simulink model "BANSHEE"  (Simulink 8.7)
settings: Solver=ode1  StartTime=0.0  StopTime=inf  FixedStep=Ts  MaxStep=1e-3  RelTol=1e-3
PostLoadFcn:
  | BANSHEE_init;
InitFcn:
  | BANSHEE_init;
values from neighbouring files (symbols this model uses):
  Ts = 100E-6    (= 0.0001)    [BANSHEE_init.m]
undefined symbols (not defined in the file or in its folder): Acid, Banshee_HWCtrl_IOs, Banshee_SEL751_Woodward_lib, DMS_slave_lib, DMSCommands, F1, F2, F3, fdesignblkfcn, Feeder1_lib, Feeder2_lib, Feeder3_lib, gcbh, generic_ethernet_cb, Lead, Left, relay_housing_lib, SM_UtilityService, SS_F1_RELAY_HOUSING, SS_F2_RELAY_HOUSING, SS_F3_RELAY_HOUSING, SS_Feeder1, SS_Feeder2, SS_Feeder3, SUBSTATION, TestSeq_slave_lib, TestSequenceCommands, type, utility_service_lib, V
libraries: powerlib x108, cables_lib x61, breaker_lib x53, rtio_generic_modbus x50, relay_modbus_lib x45, rtio_opalrt_op5142ex1 x37, transformer_lib x29, rteventslib x28, Load_lib x25, simulink x24, rtlab x20, ssn_lib x19
(part 4 of 9)

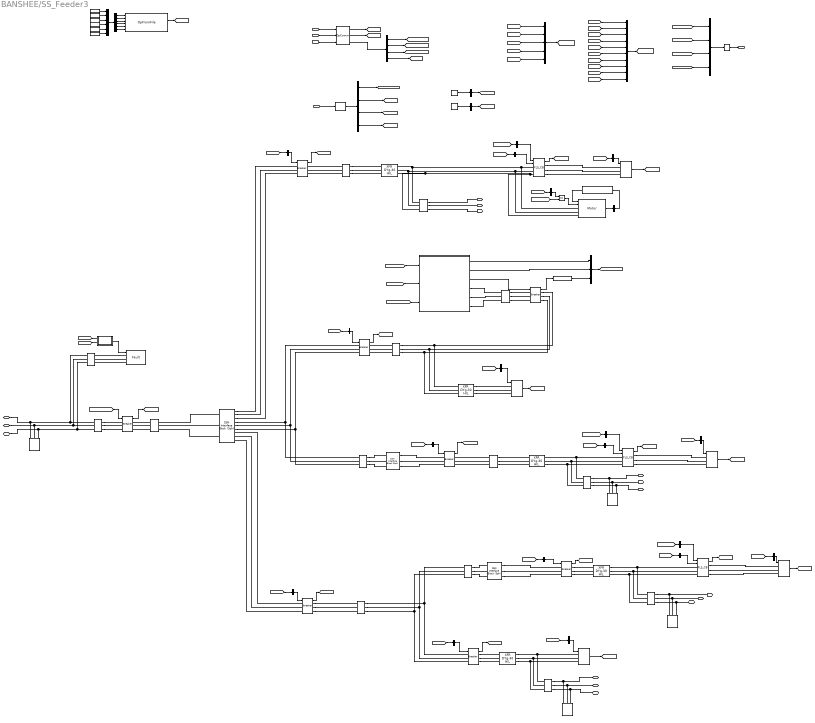
== system BANSHEE/SS_Feeder3 ==
  note: Signal for this Cb will come from a SEL relay
  note: connect to F2
  note: connect to F2
  note: connect to F2
  note: connect to F1
  note: % Copyright (c) 2016 Massachusetts Institute of Technology
      | % Permission is hereby granted, free of charge, to any person obtaining a copy of this
      | % software and associated documentation files (the "Software"), to deal in the Software
      | % without restriction, including without limitation the rights to use, copy, modify,
      | % merge, publish, distribute, sublicense, and/or sell copies of the Software, and to
      | % permit persons to whom the Software is furnished to do so, subject to the following
      | % conditions:
      | %
      | %
      | % The above copyright notice and this permission notice shall be included in
      | % all copies or substantial portions of the Software.
      | %
      | % THE SOFTWARE IS PROVIDED "AS IS", WITHOUT WARRANTY OF ANY KIND, EXPRESS OR IMPLIED,
      | % INCLUDING BUT NOT LIMITED TO THE WARRANTIES OF MERCHANTABILITY, FITNESS FOR A
      | % PARTICULAR PURPOSE AND NONINFRINGEMENT. IN NO EVENT SHALL THE AUTHORS OR COPYRIGHT
      | % HOLDERS BE LIABLE FOR ANY CLAIM, DAMAGES OR OTHER LIABILITY, WHETHER IN AN ACTION
      | % OF CONTRACT, TORT OR OTHERWISE, ARISING FROM, OUT OF OR IN CONNECTION WITH THE
      | % SOFTWARE OR THE USE OR OTHER DEALINGS IN THE SOFTWARE.
      | %
      | %
      | %%
  RELAY_IN : Inport
  LOAD_IN : Inport  Port=2
  SC_CMD : Inport  Port=3
  HWCtrl_CMD : Inport  Port=4
  1000 kVA : transformer_lib/XFR DYg-30 HIL  Rating=1000  Vp=13800  Vs=480  Z=5.75  XR=4.21
  1000 kVA1 : transformer_lib/XFR DYg-30 HIL  Rating=1000  Vp=13800  Vs=480  Z=5.75  XR=4.21
  200 HP chiller compressor : Load_lib/200 HP chiller compressor
  2000 kVA : transformer_lib/XFR DYg-30 HIL  Rating=2000  Vp=13800  Vs=480  Z=5.75  XR=4.7
  2000 kVA1 : transformer_lib/XFR DYg-30 HIL  Rating=2000  Vp=13800  Vs=480  Z=5.75  XR=4.7
  2500 kVA : transformer_lib/XFR DYg-30 HIL  Rating=2500  Vp=13800  Vs=480  Z=5.75  XR=6.6
  4/0AWG-Mutual : cables_lib/4//0AWG-Mutual  length=100  par_sets=1  ratio=3
  448 kvar inductor at 13.8kV  to cancel kvar produced by the stublines1 : powerlib/Elements/Three-Phase Parallel RLC Load  LConnTagsString=A|B|C  Configuration=Y (grounded)  NominalVoltage=13800  Vabc=[1e3 1e3 1e3]  Vabcp=[1e3 1e3 1e3]  NominalFrequency=60  UnbalancedPower=off  ActivePower=0  InductivePower=448e3  CapacitivePower=0  Pabc=[10e3 9e3 11e3]  QLabc=[100 90 110]  QCabc=[100 90 110]  Pabcp=[10e3 9e3 11e3]  QLabcp=[100 90 110]  QCabcp=[100 90 110]  Measurements=None  LoadType=constant Z
  500kcmil-Mutual{1..2,4,7} (4 alike) : cables_lib/500kcmil-Mutual  length=10  par_sets=1  ratio=3
  500kcmil-Mutual3 : cables_lib/500kcmil-Mutual  length=100  par_sets=1  ratio=3
  500kcmil-Mutual5 : cables_lib/500kcmil-Mutual  length=1000  par_sets=1  ratio=3
  500kcmil-Mutual9 : cables_lib/500kcmil-Mutual  length=1  par_sets=1  ratio=3
  6 kvar inductor at 480V  to cancel kvar produced by the stublines1 : powerlib/Elements/Three-Phase Parallel RLC Load  LConnTagsString=A|B|C  Configuration=Y (grounded)  NominalVoltage=480  Vabc=[1e3 1e3 1e3]  Vabcp=[1e3 1e3 1e3]  NominalFrequency=60  UnbalancedPower=off  ActivePower=0  InductivePower=6e3  CapacitivePower=0  Pabc=[10e3 9e3 11e3]  QLabc=[100 90 110]  QCabc=[100 90 110]  Pabcp=[10e3 9e3 11e3]  QLabcp=[100 90 110]  QCabcp=[100 90 110]  Measurements=None  LoadType=constant Z
  6 kvar inductor at 480V  to cancel kvar produced by the stublines2 : powerlib/Elements/Three-Phase Parallel RLC Load  LConnTagsString=A|B|C  Configuration=Y (grounded)  NominalVoltage=480  Vabc=[1e3 1e3 1e3]  Vabcp=[1e3 1e3 1e3]  NominalFrequency=60  UnbalancedPower=off  ActivePower=0  InductivePower=6e3  CapacitivePower=0  Pabc=[10e3 9e3 11e3]  QLabc=[100 90 110]  QCabc=[100 90 110]  Pabcp=[10e3 9e3 11e3]  QLabcp=[100 90 110]  QCabcp=[100 90 110]  Measurements=None  LoadType=constant Z
  6 kvar inductor at 480V  to cancel kvar produced by the stublines3 : powerlib/Elements/Three-Phase Parallel RLC Load  LConnTagsString=A|B|C  Configuration=Y (grounded)  NominalVoltage=480  Vabc=[1e3 1e3 1e3]  Vabcp=[1e3 1e3 1e3]  NominalFrequency=60  UnbalancedPower=off  ActivePower=0  InductivePower=6e3  CapacitivePower=0  Pabc=[10e3 9e3 11e3]  QLabc=[100 90 110]  QCabc=[100 90 110]  Pabcp=[10e3 9e3 11e3]  QLabcp=[100 90 110]  QCabcp=[100 90 110]  Measurements=None  LoadType=constant Z
  Bus Creator : BusCreator  Inputs=1
  Bus Creator1 : BusCreator  Inputs=1
  Bus Creator2 : BusCreator  Inputs=4
  Bus Creator3 : BusCreator  Inputs=5
  Bus Creator5 : BusCreator  Inputs=10
  Bus Creator6 : BusCreator  Inputs=3
  Bus Selector : BusSelector  OutputSignals=motor_2
  Bus Selector1 : BusSelector  OutputSignals=F3_CB_4
  Bus Selector10 : BusSelector  OutputSignals=F3_CB_5
  Bus Selector11 : BusSelector  OutputSignals=P6
  Bus Selector12 : BusSelector  OutputSignals=F3_CB_9
  Bus Selector13 : BusSelector  OutputSignals=F3_CB_3
  Bus Selector14 : BusSelector  OutputSignals=F3_CB_8
  Bus Selector15 : BusSelector  OutputSignals=IO ctrl.16 DOUT GR3.CHP_SIM_Cmds,motor_ONOFF.F3_motor_ONOFF,fault_cmd,GridStatusCtrl.Grid_F3.Logic_trip
  Bus Selector16 : BusSelector  OutputSignals=HWCtrl.NGCHP_Gen1,HWCtrl.SEL751_LogicTrip.F3.Logic_trip,HWCtrl.SEL2440_FLS,TestSeq
  Bus Selector17 : BusSelector  OutputSignals=RPM
  Bus Selector18 : BusSelector  OutputSignals=CB309
  Bus Selector19 : BusSelector  OutputSignals=CB307
  Bus Selector2 : BusSelector  OutputSignals=C6
  Bus Selector20 : BusSelector  OutputSignals=CB308
  Bus Selector3 : BusSelector  OutputSignals=P4
  Bus Selector4 : BusSelector  OutputSignals=I6
  Bus Selector5 : BusSelector  OutputSignals=C5
  Bus Selector6 : BusSelector  OutputSignals=F3_CB_2
  Bus Selector7 : BusSelector  OutputSignals=F3_CB_7
  Bus Selector8 : BusSelector  OutputSignals=F3_CB_6
  Bus Selector9 : BusSelector  OutputSignals=F3_CB_1
  C1 : cables_lib/500kcmil-Mutual  length=10  par_sets=1  ratio=3
  C2 : cables_lib/500kcmil-Mutual  length=10  par_sets=1  ratio=3
  C301 : cables_lib/500kcmil-Mutual  length=2500  par_sets=1  ratio=3
  C302 : cables_lib/4//0AWG-Mutual  length=2000  par_sets=1  ratio=3
  C303 : cables_lib/500kcmil-Mutual  length=2000  par_sets=1  ratio=3
  C304 : cables_lib/4//0AWG-Mutual  length=1500  par_sets=2  ratio=3
  CB closed : Constant
  CB open : Constant  Value=0
  Critical_5 : Load_lib/Dynamic_Load  V=480  kVA=1000  PF=0.9  Ts=Ts
  Critical_6 : Load_lib/Dynamic_Load  V=480  kVA=800  PF=0.9  Ts=Ts
  Demux2 : Demux  Outputs=6
  F3_CB_{1..6} (6 alike) : breaker_lib/Breaker  Ts=Ts  mech_delay=cb_mech_delay
  F3_CB_7 : breaker_lib/FLS_CB  Ts=Ts  mech_delay=cb_mech_delay
  F3_CB_8 : breaker_lib/FLS_CB  Ts=Ts  mech_delay=cb_mech_delay
  F3_CB_9 : breaker_lib/FLS_CB  Ts=Ts  mech_delay=cb_mech_delay
  F3_GCB : breaker_lib/Breaker  Ts=Ts  mech_delay=cb_mech_delay
  F3_PCC : breaker_lib/Breaker  Ts=Ts  mech_delay=cb_mech_delay
  Fault_4 : fault_lib/Fault  FaultResistance=0.1  GroundResistance=0.01  SnubberResistance=1E6
  HWController_3.5MVA_NGCHP : Subsystem  AncestorBlock=HWController_NGCHP_Genset_3p5MVA_lib/HWController_3.5MVA_NGCHP
  "Interpolation " : Constant
  Interruptible_6 : Load_lib/Dynamic_Load  V=480  kVA=600  PF=0.9  Ts=Ts
  Logical Operator : Logic  Operator=OR  AllPortsSameDT=off  OutDataTypeStr=boolean
  Memory : Memory
  Motor : Motor_InductionMachine_lib/Motor
  Mux : Mux  Inputs=6
  OpComm1 : rtlab/OpComm  nbport=3  groupe_acq=1  subsys_rate=0  st=0  Synchronization=on  Interpolation=on  Threshold=1.0  Missed_Data=off  Sim_Time=off  Samples=off  dynSigOut=off  from_console=0  warning_done=off  writeOpCommFile=off  Offset=off
  OpComm2 : rtlab/OpComm  nbport=1  groupe_acq=1  subsys_rate=0  st=0  Synchronization=on  Interpolation=on  Threshold=1.0  Missed_Data=off  Sim_Time=off  Samples=off  dynSigOut=off  from_console=1  warning_done=off  writeOpCommFile=off  Offset=off
  OpFromFile : rtlab/DataLogging/OpFromFile  filename_mode=Static (same filename all the time)  reload_mode=Next time model is paused (Real-Time)  init_file_id=0  filename=HeatLoad.mat  rtpath='./'  nrtpath='.\'  sample_time=Ts
  PQFV : PQFV_lib/PQFV  VRMSLL=13800  Ts=Ts
  Priority_4 : Load_lib/Dynamic_Load  V=480  kVA=600  PF=0.9  Ts=Ts
  Priority_6 : Load_lib/Dynamic_Load  V=480  kVA=1000  PF=0.9  Ts=Ts
  "Repetative " : Constant
  SSN Interface Block (3ph)1 : ssn_lib/SSN Interface Block (3ph)  nb_phase=3  nb_port=2  p1_type=V-type(Left)  p2_type=V-type (Right)  p3_type=V-type(Left)  p4_type=V-type(Left)  p5_type=V-type(Left)  p6_type=V-type(Left)  p7_type=V-type(Left)  p8_type=V-type(Left)  p9_type=V-type(Left)  p10_type=V-type(Left)  p11_type=V-type(Left)  p12_type=V-type(Left)  p13_type=V-type(Left)  p14_type=V-type(Left)  p15_type=V-type(Left)  p16_type=V-type(Left)  I_port_shunt_resistance=1e9
  SSN Interface Block (3ph)2 : ssn_lib/SSN Interface Block (3ph)  nb_phase=3  nb_port=2  p1_type=V-type(Left)  p2_type=V-type (Right)  p3_type=V-type(Left)  p4_type=V-type(Left)  p5_type=V-type(Left)  p6_type=V-type(Left)  p7_type=V-type(Left)  p8_type=V-type(Left)  p9_type=V-type(Left)  p10_type=V-type(Left)  p11_type=V-type(Left)  p12_type=V-type(Left)  p13_type=V-type(Left)  p14_type=V-type(Left)  p15_type=V-type(Left)  p16_type=V-type(Left)  I_port_shunt_resistance=1e9
  SSN Interface Block (3ph)5 : ssn_lib/SSN Interface Block (3ph)  nb_phase=3  nb_port=4  p1_type=V-type(Left)  p2_type=V-type (Right)  p3_type=V-type (Right)  p4_type=V-type (Right)  p5_type=V-type(Left)  p6_type=V-type(Left)  p7_type=V-type(Left)  p8_type=V-type(Left)  p9_type=V-type(Left)  p10_type=V-type(Left)  p11_type=V-type(Left)  p12_type=V-type(Left)  p13_type=V-type(Left)  p14_type=V-type(Left)  p15_type=V-type(Left)  p16_type=V-type(Left)  I_port_shunt_resistance=1e9
  "Start_Index " : Constant
  "State " : Constant
  "Stop_Index " : Constant  Value=1800-1
  "Time_Scale_Factor " : Constant
  fault_signal : Subsystem
  A_CB_4 : PMIOPort  Port=1  Side=Right
  B_CB_4 : PMIOPort  Port=2  Side=Right
  C_CB_4 : PMIOPort  Port=3  Side=Right
  A_CB_5 : PMIOPort  Port=4  Side=Right
  B_CB_5 : PMIOPort  Port=5  Side=Right
  C_CB_5 : PMIOPort  Port=6  Side=Right
  A_CB_6 : PMIOPort  Port=7  Side=Right
  B_CB_6 : PMIOPort  Port=8  Side=Right
  C_CB_6 : PMIOPort  Port=9  Side=Right
  A_CB_7 : PMIOPort  Port=10  Side=Right
  B_CB_7 : PMIOPort  Port=11  Side=Right
  C_CB_7 : PMIOPort  Port=12  Side=Right
  PCC_A : PMIOPort  Port=13  Side=Left
  PCC_B : PMIOPort  Port=14  Side=Left
  PCC_C : PMIOPort  Port=15  Side=Left
  DATA_OUT : Outport
  wires:
  CB closed/1 -> Bus Creator/1  "Logic_trip"
  Bus Creator/1 -> [cb_c]
  Bus Creator1/1 -> [cb_o]
  Bus Selector1/1 -> F3_CB_4/1  "<F3_CB_4>"
  CB open/1 -> Bus Creator1/1  "Logic_trip"
  LOAD_IN/1 -> OpComm1/1
  OpComm1/1 -> [LOAD_IN]
  [LOAD_IN] -> Bus Selector2/1
  [LOAD_IN] -> Bus Selector3/1
  [LOAD_IN] -> Bus Selector4/1
  [LOAD_IN] -> Bus Selector5/1
  Bus Selector2/1 -> Critical_6/1  "<C6>"
  Bus Selector3/1 -> Priority_4/1  "<P4>"
  Bus Selector4/1 -> Interruptible_6/1  "<I6>"
  Bus Selector5/1 -> Critical_5/1  "<C5>"
  Critical_6/1 -> [LOAD_C6]
  Priority_4/1 -> [LOAD_P4]
  Interruptible_6/1 -> [LOAD_I6]
  Critical_5/1 -> [LOAD_C5]
  [LOAD_C6] -> Bus Creator3/2  "F3_C6"
  [LOAD_C5] -> Bus Creator3/1  "F3_C5"
  [LOAD_I6] -> Bus Creator3/3  "F3_I6"
  [LOAD_P4] -> Bus Creator3/4  "F3_P4"
  Bus Creator3/1 -> [LOAD_DATA]  "LOAD"
  F3_CB_4/1 -> [F3_CB_4]
  F3_CB_3/1 -> [F3_CB_3]
  F3_CB_2/1 -> [F3_CB_2]
  F3_CB_6/1 -> [F3_CB_6]
  F3_CB_1/1 -> [F3_CB_1]
  F3_CB_5/1 -> [F3_CB_5]
  [F3_CB_1] -> Bus Creator5/1  "F3_CB_1"
  [F3_CB_5] -> Bus Creator5/5  "F3_CB_5"
  [F3_CB_7] -> Bus Creator5/7  "F3_CB_7"
  [F3_CB_6] -> Bus Creator5/6  "F3_CB_6"
  [F3_CB_3] -> Bus Creator5/3  "F3_CB_3"
  [F3_CB_2] -> Bus Creator5/2  "F3_CB_2"
  [F3_CB_4] -> Bus Creator5/4  "F3_CB_4"
  Bus Creator5/1 -> [CB_DATA]
  [RELAY_IN] -> Bus Selector1/1
  RELAY_IN/1 -> OpComm1/2
  OpComm1/2 -> [RELAY_IN]
  Bus Selector6/1 -> F3_CB_2/1  "<F3_CB_2>"
  [RELAY_IN] -> Bus Selector6/1
  Bus Selector7/1 -> F3_CB_7/2  "<F3_CB_7>"
  [RELAY_IN] -> Bus Selector7/1
  Bus Selector8/1 -> F3_CB_6/1  "<F3_CB_6>"
  [RELAY_IN] -> Bus Selector8/1
  Bus Selector9/1 -> F3_CB_1/1  "<F3_CB_1>"
  [RELAY_IN] -> Bus Selector9/1
  Bus Selector10/1 -> F3_CB_5/1  "<F3_CB_5>"
  [RELAY_IN] -> Bus Selector10/1
  Bus Selector13/1 -> F3_CB_3/1  "<F3_CB_3>"
  [RELAY_IN] -> Bus Selector13/1
  [SEL751_F3_LogicTrip] -> F3_PCC/1
  F3_CB_7/1 -> [F3_CB_7]
  F3_PCC/1 -> [F3_PCC]
  [F3_PCC] -> Bus Creator5/10  "F3_PCC"
  [LOAD_IN] -> Bus Selector11/1
  Bus Selector11/1 -> Priority_6/1  "<P6>"
  Priority_6/1 -> [LOAD_P6]
  [LOAD_P6] -> Bus Creator3/5  "F3_P6"
  F3_CB_9/1 -> [F3_CB_9]
  Bus Selector12/1 -> F3_CB_9/2  "<F3_CB_9>"
  [RELAY_IN] -> Bus Selector12/1
  F3_CB_8/1 -> [F3_CB_8]
  Bus Selector14/1 -> F3_CB_8/2  "<F3_CB_8>"
  [RELAY_IN] -> Bus Selector14/1
  [F3_CB_8] -> Bus Creator5/8  "F3_CB_8"
  [F3_CB_9] -> Bus Creator5/9  "F3_CB_9"
  SC_CMD/1 -> OpComm2/1
  Memory/1 -> DATA_OUT/1
  "Start_Index "/1 -> Mux/3
  "Time_Scale_Factor "/1 -> Mux/5
  "State "/1 -> Mux/1
  Demux2/1 -> OpFromFile/1
  Demux2/4 -> OpFromFile/4
  OpFromFile/2 -> [heat_load]  "Heat Load MBtu/hr"
  Demux2/5 -> OpFromFile/5
  "Repetative "/1 -> Mux/2
  Demux2/3 -> OpFromFile/3
  Demux2/6 -> OpFromFile/6
  Demux2/2 -> OpFromFile/2
  Mux/1 -> Demux2/1
  "Interpolation "/1 -> Mux/6
  "Stop_Index "/1 -> Mux/4
  Bus Selector15/2 -> [motor_cmd]  "<F3_motor_ONOFF>"
  OpComm2/1 -> Bus Selector15/1
  Bus Selector15/3 -> [fault_cmd]  "<fault_cmd>"
  F3_GCB/1 -> PQFV/1
  PQFV/1 -> Bus Creator6/3  "NG_CHP_GCB"
  HWController_3.5MVA_NGCHP/2(Generator Data) -> Bus Creator6/2  "Gen1_meas"
  HWController_3.5MVA_NGCHP/1(Out1) -> Bus Creator6/1  "CHPData"
  [CHP_SIM_cmds] -> HWController_3.5MVA_NGCHP/2(In2)
  Bus Creator6/1 -> [NG_CHP_DATA]
  [NGCHP_Gen1] -> HWController_3.5MVA_NGCHP/3(HWControllerBias)
  HWController_3.5MVA_NGCHP/3(GCB Control) -> F3_GCB/1
  [heat_load] -> HWController_3.5MVA_NGCHP/1(Heat Load MBtu/hrs)
  HWCtrl_CMD/1 -> OpComm1/3
  OpComm1/3 -> Bus Selector16/1
  Bus Selector16/1 -> [NGCHP_Gen1]  "<NGCHP_Gen1>"
  Bus Creator2/1 -> Memory/1
  [CB_DATA] -> Bus Creator2/1  "CB_DATA"
  [LOAD_DATA] -> Bus Creator2/2  "LOAD_DATA"
  [NG_CHP_DATA] -> Bus Creator2/3  "NG_CHP_DATA"
  Bus Selector15/1 -> [CHP_SIM_cmds]  "<CHP_SIM_Cmds>"
  Motor/1 -> Bus Selector17/1
  Bus Selector17/1 -> 200 HP chiller compressor/1  "<RPM>"
  200 HP chiller compressor/1 -> Motor/1
  [motor_cmd] -> Bus Creator2/4  "MOTOR_ONOFF"
  Bus Selector16/2 -> [SEL751_F3_LogicTrip]  "<Logic_trip>"
  Bus Selector16/3 -> [SEL_2440_FLS]  "<SEL2440_FLS>"
  [SEL_2440_FLS] -> Bus Selector18/1
  Bus Selector18/1 -> F3_CB_9/1  "<CB309>"
  [SEL_2440_FLS] -> Bus Selector19/1
  Bus Selector19/1 -> F3_CB_7/1  "<CB307>"
  [SEL_2440_FLS] -> Bus Selector20/1
  Bus Selector20/1 -> F3_CB_8/1  "<CB308>"
  Bus Selector15/4 -> [feeder_cb]  "<Logic_trip>"
  Bus Selector16/4 -> [TestSeq]  "<TestSeq>"
  [TestSeq] -> fault_signal/1(fault_ts)
  [fault_cmd] -> fault_signal/2(fault_sc)
  fault_signal/1(o) -> Fault_4/1
  [TestSeq] -> Bus Selector/1
  Logical Operator/1 -> Motor/2
  Bus Selector/1 -> Logical Operator/1  "<motor_2>"
  [motor_cmd] -> Logical Operator/2
  connections:
  C301/RConn1 -- C1/LConn1 -- F3_CB_5/LConn1
  F3_CB_6/RConn3 -- 2000 kVA1/LConn3
  C301/RConn3 -- C1/LConn3 -- F3_CB_5/LConn3
  C304/LConn1 -- F3_CB_2/RConn1
  F3_GCB/RConn3 -- C302/RConn3 -- 1000 kVA1/LConn3
  C302/LConn2 -- F3_CB_3/RConn2
  F3_GCB/RConn1 -- C302/RConn1 -- 1000 kVA1/LConn1
  F3_CB_6/RConn2 -- 2000 kVA1/LConn2
  F3_GCB/RConn2 -- C302/RConn2 -- 1000 kVA1/LConn2
  F3_CB_5/RConn2 -- 2000 kVA/LConn2
  C302/LConn3 -- F3_CB_3/RConn3
  C301/RConn2 -- C1/LConn2 -- F3_CB_5/LConn2
  C304/LConn2 -- F3_CB_2/RConn2
  F3_CB_6/RConn1 -- 2000 kVA1/LConn1
  C302/LConn1 -- F3_CB_3/RConn1
  F3_CB_5/RConn1 -- 2000 kVA/LConn1
  F3_CB_5/RConn3 -- 2000 kVA/LConn3
  C304/LConn3 -- F3_CB_2/RConn3
  F3_CB_7/RConn1 -- Priority_4/LConn1
  F3_CB_7/RConn3 -- Priority_4/LConn3
  F3_CB_7/RConn2 -- Priority_4/LConn2
  2000 kVA1/RConn1 -- 500kcmil-Mutual2/LConn1 -- F3_CB_8/LConn1
  500kcmil-Mutual2/LConn3 -- F3_CB_8/LConn3 -- 2000 kVA1/RConn3
  2000 kVA1/RConn2 -- 500kcmil-Mutual2/LConn2 -- F3_CB_8/LConn2
  2000 kVA/RConn1 -- 500kcmil-Mutual1/LConn1 -- Critical_5/LConn1
  2000 kVA/RConn3 -- 500kcmil-Mutual1/LConn3 -- Critical_5/LConn3
  2000 kVA/RConn2 -- 500kcmil-Mutual1/LConn2 -- Critical_5/LConn2
  Motor/LConn1 -- F3_CB_9/LConn1 -- 500kcmil-Mutual9/LConn1 -- 2500 kVA/RConn1
  F3_CB_9/LConn3 -- Motor/LConn3 -- 500kcmil-Mutual9/LConn3 -- 2500 kVA/RConn3
  Motor/LConn2 -- F3_CB_9/LConn2 -- 500kcmil-Mutual9/LConn2 -- 2500 kVA/RConn2
  C304/RConn2 -- 1000 kVA/LConn2
  C304/RConn3 -- 1000 kVA/LConn3
  C304/RConn1 -- 1000 kVA/LConn1
  F3_CB_7/LConn2 -- 500kcmil-Mutual4/LConn2 -- 1000 kVA/RConn2
  F3_CB_7/LConn1 -- 500kcmil-Mutual4/LConn1 -- 1000 kVA/RConn1
  F3_CB_9/RConn1 -- Priority_6/LConn1
  F3_CB_9/RConn2 -- Priority_6/LConn2
  F3_CB_9/RConn3 -- Priority_6/LConn3
  F3_CB_8/RConn1 -- Interruptible_6/LConn1
  F3_CB_8/RConn2 -- Interruptible_6/LConn2
  F3_CB_8/RConn3 -- Interruptible_6/LConn3
  SSN Interface Block (3ph)5/RConn1 -- F3_CB_4/LConn1
  SSN Interface Block (3ph)5/RConn3 -- F3_CB_4/LConn3
  SSN Interface Block (3ph)5/RConn2 -- F3_CB_4/LConn2
  SSN Interface Block (3ph)5/RConn4 -- F3_CB_3/LConn1 -- C2/LConn1
  SSN Interface Block (3ph)5/RConn6 -- F3_CB_3/LConn3 -- C2/LConn3
  SSN Interface Block (3ph)5/RConn5 -- C2/LConn2 -- F3_CB_3/LConn2
  C303/LConn1 -- F3_CB_4/RConn1
  C303/LConn2 -- F3_CB_4/RConn2
  C303/LConn3 -- F3_CB_4/RConn3
  C303/RConn2 -- 2500 kVA/LConn2
  C303/RConn3 -- 2500 kVA/LConn3
  C303/RConn1 -- 2500 kVA/LConn1
  Fault_4/LConn2 -- 500kcmil-Mutual7/RConn2
  Fault_4/LConn3 -- 500kcmil-Mutual7/RConn3
  Fault_4/LConn1 -- 500kcmil-Mutual7/RConn1
  4/0AWG-Mutual/RConn3 -- F3_GCB/LConn3
  4/0AWG-Mutual/RConn2 -- F3_GCB/LConn2
  4/0AWG-Mutual/RConn1 -- F3_GCB/LConn1
  HWController_3.5MVA_NGCHP/RConn2 -- 4/0AWG-Mutual/LConn2
  HWController_3.5MVA_NGCHP/RConn3 -- 4/0AWG-Mutual/LConn3
  HWController_3.5MVA_NGCHP/RConn1 -- 4/0AWG-Mutual/LConn1
  1000 kVA1/RConn1 -- Critical_6/LConn1
  1000 kVA1/RConn2 -- Critical_6/LConn2
  1000 kVA1/RConn3 -- Critical_6/LConn3
  500kcmil-Mutual1/RConn2 -- B_CB_5/RConn1 -- 6 kvar inductor at 480V  to cancel kvar produced by the stublines2/LConn2
  500kcmil-Mutual1/RConn1 -- 6 kvar inductor at 480V  to cancel kvar produced by the stublines2/LConn1 -- A_CB_5/RConn1
  500kcmil-Mutual1/RConn3 -- C_CB_5/RConn1 -- 6 kvar inductor at 480V  to cancel kvar produced by the stublines2/LConn3
  500kcmil-Mutual2/RConn2 -- 6 kvar inductor at 480V  to cancel kvar produced by the stublines1/LConn2 -- B_CB_6/RConn1
  500kcmil-Mutual2/RConn3 -- 6 kvar inductor at 480V  to cancel kvar produced by the stublines1/LConn3 -- C_CB_6/RConn1
  500kcmil-Mutual2/RConn1 -- 6 kvar inductor at 480V  to cancel kvar produced by the stublines1/LConn1 -- A_CB_6/RConn1
  500kcmil-Mutual4/RConn2 -- 6 kvar inductor at 480V  to cancel kvar produced by the stublines3/LConn2 -- B_CB_7/RConn1
  500kcmil-Mutual4/RConn3 -- 6 kvar inductor at 480V  to cancel kvar produced by the stublines3/LConn3 -- C_CB_7/RConn1
  500kcmil-Mutual4/RConn1 -- A_CB_7/RConn1 -- 6 kvar inductor at 480V  to cancel kvar produced by the stublines3/LConn1
  500kcmil-Mutual9/RConn1 -- A_CB_4/RConn1
  500kcmil-Mutual9/RConn3 -- C_CB_4/RConn1
  500kcmil-Mutual9/RConn2 -- B_CB_4/RConn1
  500kcmil-Mutual3/LConn3 -- F3_PCC/RConn3
  500kcmil-Mutual3/LConn1 -- F3_PCC/RConn1
  500kcmil-Mutual3/LConn2 -- F3_PCC/RConn2
  500kcmil-Mutual5/RConn1 -- F3_PCC/LConn1
  500kcmil-Mutual5/RConn2 -- F3_PCC/LConn2
  500kcmil-Mutual5/RConn3 -- F3_PCC/LConn3
  1000 kVA/RConn3 -- 500kcmil-Mutual4/LConn3 -- F3_CB_7/LConn3
  C1/RConn2 -- SSN Interface Block (3ph)1/LConn2
  C1/RConn3 -- SSN Interface Block (3ph)1/LConn3
  C1/RConn1 -- SSN Interface Block (3ph)1/LConn1
  SSN Interface Block (3ph)5/LConn1 -- 500kcmil-Mutual3/RConn1
  SSN Interface Block (3ph)5/LConn2 -- 500kcmil-Mutual3/RConn2
  SSN Interface Block (3ph)5/LConn3 -- 500kcmil-Mutual3/RConn3
  PCC_A/RConn1 -- 500kcmil-Mutual7/LConn1 -- 500kcmil-Mutual5/LConn1 -- 448 kvar inductor at 13.8kV  to cancel kvar produced by the stublines1/LConn1
  PCC_B/RConn1 -- 448 kvar inductor at 13.8kV  to cancel kvar produced by the stublines1/LConn2 -- 500kcmil-Mutual7/LConn2 -- 500kcmil-Mutual5/LConn2
  PCC_C/RConn1 -- 448 kvar inductor at 13.8kV  to cancel kvar produced by the stublines1/LConn3 -- 500kcmil-Mutual7/LConn3 -- 500kcmil-Mutual5/LConn3
  SSN Interface Block (3ph)2/RConn3 -- F3_CB_2/LConn3
  SSN Interface Block (3ph)2/RConn2 -- F3_CB_2/LConn2
  SSN Interface Block (3ph)2/RConn1 -- F3_CB_2/LConn1
  C2/RConn2 -- SSN Interface Block (3ph)2/LConn2
  C2/RConn1 -- SSN Interface Block (3ph)2/LConn1
  C2/RConn3 -- SSN Interface Block (3ph)2/LConn3
  F3_CB_1/LConn2 -- SSN Interface Block (3ph)5/RConn8
  F3_CB_1/LConn1 -- SSN Interface Block (3ph)5/RConn7
  F3_CB_1/LConn3 -- SSN Interface Block (3ph)5/RConn9
  SSN Interface Block (3ph)1/RConn1 -- F3_CB_6/LConn1
  SSN Interface Block (3ph)1/RConn2 -- F3_CB_6/LConn2
  SSN Interface Block (3ph)1/RConn3 -- F3_CB_6/LConn3
  F3_CB_1/RConn1 -- C301/LConn1
  F3_CB_1/RConn2 -- C301/LConn2
  F3_CB_1/RConn3 -- C301/LConn3

== system BANSHEE/SS_PV_BESS ==
  SC_CMD : Inport
  25% : Load_lib/Series_Constant_Load  v=480  kVA=1000  pf=0.9
  BESS : BESS_lib/BESS
  BESS Measurements : Subsystem
  Bus Creator6 : BusCreator  Inputs=2
  Bus Selector7 : BusSelector  OutputSignals=SWR_BESS,EPC_CTRL
  C1 : cables_lib/500kcmil-Mutual  length=10  par_sets=1  ratio=3
  C2 : cables_lib/500kcmil-Mutual  length=10  par_sets=1  ratio=3
  EPC : Subsystem
  Memory : Memory
  OpComm3 : rtlab/OpComm  nbport=1  groupe_acq=1  subsys_rate=0  st=0  Synchronization=on  Interpolation=on  Threshold=1.0  Missed_Data=off  Sim_Time=off  Samples=off  dynSigOut=off  from_console=1  warning_done=off  writeOpCommFile=off  Offset=off
  PV Measurements : Subsystem
  A_PV : PMIOPort  Port=1  Side=Right
  B_PV : PMIOPort  Port=2  Side=Right
  C_PV : PMIOPort  Port=3  Side=Right
  A_BESS : PMIOPort  Port=4  Side=Right
  B_BESS : PMIOPort  Port=5  Side=Right
  C_BESS : PMIOPort  Port=6  Side=Right
  BESS_PV : Outport
  wires:
  SC_CMD/1 -> OpComm3/1
  OpComm3/1 -> Bus Selector7/1
  Bus Selector7/1 -> [SWR_BESS]  "<SWR_BESS>"
  [SWR_BESS] -> BESS/1
  BESS/1 -> [BESS_MS]
  Memory/1 -> BESS_PV/1
  Bus Creator6/1 -> Memory/1
  [BESS_MS] -> Bus Creator6/1  "BESS"
  EPC/1(monitoring) -> [EPC_MS]
  [EPC_MS] -> Bus Creator6/2  "EPC"
  Bus Selector7/2 -> [EPC_CTRL]  "<EPC_CTRL>"
  [EPC_CTRL] -> EPC/1(FROM_SC)
  [EPC_MS] -> BESS Measurements/1(EPC_MS)
  [EPC_MS] -> PV Measurements/1(EPC_MS)
  connections:
  B_BESS/RConn1 -- C1/RConn2
  C_BESS/RConn1 -- C1/RConn3
  A_BESS/RConn1 -- C1/RConn1
  B_PV/RConn1 -- C2/RConn2
  C_PV/RConn1 -- C2/RConn3
  A_PV/RConn1 -- C2/RConn1
  EPC/LConn1 -- C1/LConn1
  EPC/LConn2 -- C1/LConn2
  EPC/LConn3 -- C1/LConn3
  EPC/LConn5 -- C2/LConn2
  EPC/LConn4 -- C2/LConn1
  EPC/LConn6 -- C2/LConn3
  25%/LConn2 -- BESS/RConn2
  25%/LConn3 -- BESS/RConn3
  25%/LConn1 -- BESS/RConn1

== system BANSHEE/SC_ctrl/EPC Inverter ==
  note: This corresponds to
      | the DIO Enable MCB
  note: Op_Mode:
      | 0 = Relay Functions
      | 1 = Close Breaker
      | 2 = Open Breaker
  16Din/16Dout GR3 : Subsystem
  16PWMIn/16PWMout GR3 : Subsystem
  16TSDIn/16 TSDOut GR3 : Subsystem
  Brk1 Grid : Constant  Value=2
  Brk10 Gen 1 Busbar : Constant
  Brk2 Load 1 : Constant  Value=0
  Brk3 Inv MX1 : Constant  Value=2
  Brk4 Gen 1 MCB : Constant  Value=2
  Brk5 Gen 2 LCB : Constant  Value=0
  Brk6 Gen 1 LCB : Constant  Value=0
  Brk7 Gen 2 GCB : Constant
  Brk8 Gen 1 GCB : Constant
  Brk9 Gen 2 Busbar : Constant
  Bus Creator1 : BusCreator  Inputs=3
  Bus Creator2 : BusCreator  Inputs=2
  Bus Creator3 : BusCreator  Inputs=14
  Wood MCB Enable : Constant  Value=0
  bias_ctrl : Constant
  control_mode : Constant
  gen_enable : Constant
  Out1 : Outport
  wires:
  Brk10 Gen 1 Busbar/1 -> Bus Creator3/10  "Gen1_Busbar"
  Brk9 Gen 2 Busbar/1 -> Bus Creator3/9  "Gen2_Busbar"
  Brk8 Gen 1 GCB/1 -> Bus Creator3/8  "Gen1_GCB"
  Brk7 Gen 2 GCB/1 -> Bus Creator3/7  "Gen2_GCB"
  Brk6 Gen 1 LCB/1 -> Bus Creator3/6  "Load 3"
  Brk5 Gen 2 LCB/1 -> Bus Creator3/5  "Load 2"
  Wood MCB Enable/1 -> Bus Creator3/14  "Wood_MCB_enable"
  Bus Creator2/1 -> Out1/1
  bias_ctrl/1 -> Bus Creator3/13  "Gen_bias_enable"
  gen_enable/1 -> Bus Creator3/12  "Gen2_enable"
  control_mode/1 -> Bus Creator3/11  "Wood_DIO"
  Brk4 Gen 1 MCB/1 -> Bus Creator3/4  "Gen1_MCB"
  Brk3 Inv MX1/1 -> Bus Creator3/3  "MX1"
  Brk2 Load 1/1 -> Bus Creator3/2  "Load 1"
  Brk1 Grid/1 -> Bus Creator3/1  "Grid"
  Bus Creator3/1 -> Bus Creator2/2  "test_controls"
  Bus Creator1/1 -> Bus Creator2/1  "DOUT GR3"
  16PWMIn/16PWMout GR3/1(To PWMOut) -> Bus Creator1/3  "16 PWMOUT GR3"
  16TSDIn/16 TSDOut GR3/1(TSDout) -> Bus Creator1/2  "16 TSDOUT GR3"
  16Din/16Dout GR3/1(Dout) -> Bus Creator1/1  "16 DOUT GR3"

== system BANSHEE/SC_ctrl/Inv_Battery ==
  note: Make this 1 to allow
      | the external signals.
  note: Remote Sense =>1
      | Use Remote Sense EPyQ
      | Sync or not => grid forming/grid following
  note: 0=> Local
      | 1=> Remote
  note: 0=> No Console
      | 1=> Console Ctrl
  note: 1 => Sig 1 is Bot then Sig 2 is Top
      | 0 => Sig 1 is Top then Sig 2 is Bot
  note: 0=> RTE
      | 1=> Simulink
  note: LSB
  note: MSB
  note: 1111: RTE TSD Signal Modulation External
      | 0111: RTE Signal Modulation Internal
      | X011: Sin Tri Modulatiion Internal
      | XX01: Digital Inputs
      | XXX0; Open Switches
  note: MCB
  note: GCB
  note: 1 => Closed
      | 0 => Open
  note: ~ 2.5 sec to get
      | to rated voltage
  note: RTE Internal
      | All 0 and one 1
  note: Internal = 0
      | External = 1
  Bus Creator : BusCreator  Inputs=8
  Bus Creator1 : BusCreator  Inputs=5
  Console : Constant  Value=0
  DC Contactor : Constant  Value=0
  Enable PWM{0..3} (4 alike) : Constant
  MX1 : Constant  Value=0
  MX2 : Constant  Value=0
  Precharge : Constant  Value=0
  Sense : Constant  Value=0
  Signal Mapping : Constant
  Simulink : Constant  Value=0
  S : Outport
  wires:
  Sense/1 -> Bus Creator/8  "LOCALvsREMOTE"
  Console/1 -> Bus Creator/7  "Console_Ctrl"
  Signal Mapping/1 -> Bus Creator1/5  "Ext_PWM_RTE_Signal"
  Simulink/1 -> Bus Creator/6  "RTEvsSPS"
  Enable PWM3/1 -> Bus Creator1/1
  Enable PWM2/1 -> Bus Creator1/2
  Enable PWM1/1 -> Bus Creator1/3
  Enable PWM0/1 -> Bus Creator1/4
  Bus Creator1/1 -> Bus Creator/1  "Enable PWM"
  MX2/1 -> Bus Creator/5  "MX2"
  MX1/1 -> Bus Creator/4  "MX1"
  DC Contactor/1 -> Bus Creator/3  "DC_Contactor"
  Precharge/1 -> Bus Creator/2  "Precharge"
  Bus Creator/1 -> S/1

== system BANSHEE/SC_ctrl/Inv_PV ==
  note: Make this 1 to allow
      | the external signals.
  note: Remote Sense =>1
      | Use Remote Sense EPyQ
      | Sync or not => grid forming/grid following
  note: 0=> Local
      | 1=> Remote
  note: 0=> No Console
      | 1=> Console Ctrl
  note: 1 => Sig 1 is Bot then Sig 2 is Top
      | 0 => Sig 1 is Top then Sig 2 is Bot
  note: 0=> RTE
      | 1=> Simulink
  note: LSB
  note: MSB
  note: 1111: RTE TSD Signal Modulation External
      | 0111: RTE Signal Modulation Internal
      | X011: Sin Tri Modulatiion Internal
      | XX01: Digital Inputs
      | XXX0; Open Switches
  note: MCB
  note: GCB
  note: 1 => Closed
      | 0 => Open
  note: ~ 2.5 sec to get
      | to rated voltage
  note: RTE Internal
      | All 0 and one 1
  note: Internal = 0
      | External = 1
  Bus Creator : BusCreator  Inputs=8
  Bus Creator1 : BusCreator  Inputs=5
  Console : Constant  Value=0
  DC Contactor : Constant  Value=0
  Enable PWM{0..3} (4 alike) : Constant
  MX1 : Constant  Value=0
  MX2 : Constant  Value=0
  Precharge : Constant  Value=0
  Sense : Constant  Value=0
  Signal Mapping : Constant
  Simulink : Constant  Value=0
  S : Outport
  wires:
  Sense/1 -> Bus Creator/8  "LOCALvsREMOTE"
  Console/1 -> Bus Creator/7  "Console_Ctrl"
  Signal Mapping/1 -> Bus Creator1/5  "Ext_PWM_RTE_Signal"
  Simulink/1 -> Bus Creator/6  "RTEvsSPS"
  Enable PWM3/1 -> Bus Creator1/1
  Enable PWM2/1 -> Bus Creator1/2
  Enable PWM1/1 -> Bus Creator1/3
  Enable PWM0/1 -> Bus Creator1/4
  Bus Creator1/1 -> Bus Creator/1  "Enable PWM"
  MX2/1 -> Bus Creator/5  "MX2"
  MX1/1 -> Bus Creator/4  "MX1"
  DC Contactor/1 -> Bus Creator/3  "DC_Contactor"
  Precharge/1 -> Bus Creator/2  "Precharge"
  Bus Creator/1 -> S/1

== system BANSHEE/SC_ctrl/Plots ==
  note: VRMSLL
      | Hz
      | kW
      | kVAR
  CMBNE_SGNLS : Inport
  Bus Selector1 : BusSelector  OutputSignals=F1_MS_IN.DIESEL_DATA.DIESEL_GCB.VRMSLL,F1_MS_IN.DIESEL_DATA.DIESEL_GCB.Freq,F1_MS_IN.DIESEL_DATA.DIESEL_GCB.kw,F1_MS_IN.DIESEL_DATA.DIESEL_GCB.kvar  OutputAsBus=on
  Bus Selector2 : BusSelector  OutputSignals=F3_MS_IN.NG_CHP_DATA.NG_CHP_GCB.VRMSLL,F3_MS_IN.NG_CHP_DATA.NG_CHP_GCB.Freq,F3_MS_IN.NG_CHP_DATA.NG_CHP_GCB.kw,F3_MS_IN.NG_CHP_DATA.NG_CHP_GCB.kvar  OutputAsBus=on
  Bus Selector3 : BusSelector  OutputSignals=PCC_DATA_OUT.F3_PCC.VRMSLL,PCC_DATA_OUT.F3_PCC.Freq,PCC_DATA_OUT.F3_PCC.kw,PCC_DATA_OUT.F3_PCC.kvar  OutputAsBus=on
  Bus Selector4 : BusSelector  OutputSignals=PCC_DATA_OUT.F2_PCC.VRMSLL,PCC_DATA_OUT.F2_PCC.Freq,PCC_DATA_OUT.F2_PCC.kw,PCC_DATA_OUT.F2_PCC.kvar  OutputAsBus=on
  Bus Selector5 : BusSelector  OutputSignals=PCC_DATA_OUT.F1_PCC.VRMSLL,PCC_DATA_OUT.F1_PCC.Freq,PCC_DATA_OUT.F1_PCC.kw,PCC_DATA_OUT.F1_PCC.kvar  OutputAsBus=on
  Bus Selector6 : BusSelector  OutputSignals=BESS_PV.EPC.PV.PV_MX1.VRMSLL,BESS_PV.EPC.PV.PV_MX1.Freq,BESS_PV.EPC.PV.PV_MX1.kw,BESS_PV.EPC.PV.PV_MX1.kvar  OutputAsBus=on
  Bus Selector7 : BusSelector  OutputSignals=BESS_PV.EPC.BESS.BESS_MX1.VRMSLL,BESS_PV.EPC.BESS.BESS_MX1.Freq,BESS_PV.EPC.BESS.BESS_MX1.kw,BESS_PV.EPC.BESS.BESS_MX1.kvar  OutputAsBus=on
  Bus Selector8 : BusSelector  OutputSignals=BESS_PV.EPC.BESS.BESS_MX1.cb_ms.Iabc,BESS_PV.EPC.BESS.BESS_MX1.cb_ms.Vabc_line,BESS_PV.EPC.PV.PV_MX1.cb_ms.Iabc,BESS_PV.EPC.PV.PV_MX1.cb_ms.Vabc_line
  Bus Selector9 : BusSelector  OutputSignals=SUBS_RELAY_OUT.SUBSTATION_CB_F1.m.status,SUBS_RELAY_OUT.SUBSTATION_CB_F2.m.status,SUBS_RELAY_OUT.SUBSTATION_CB_F3.m.status,SUBS_RELAY_OUT.SUBSTATION_CB_F1.Logic_trip,SUBS_RELAY_OUT.SUBSTATION_CB_F2.Logic_trip,SUBS_RELAY_OUT.SUBSTATION_CB_F3.Logic_trip  OutputAsBus=on
  CHP : Display
  Diesel : Display
  EPC_BESS : Display
  EPC_PV : Display
  F1 : Display
  F2 : Display
  F3 : Display
  SUBSTATION : Display
  Scope : Scope  NumInputPorts=4
  wires:
  Bus Selector5/1 -> F1/1
  Bus Selector4/1 -> F2/1
  Bus Selector3/1 -> F3/1
  Bus Selector1/1 -> Diesel/1
  Bus Selector2/1 -> CHP/1
  CMBNE_SGNLS/1 -> [CMBNE_SGNLS]
  [CMBNE_SGNLS] -> Bus Selector5/1
  [CMBNE_SGNLS] -> Bus Selector4/1
  [CMBNE_SGNLS] -> Bus Selector3/1
  [CMBNE_SGNLS] -> Bus Selector2/1
  [CMBNE_SGNLS] -> Bus Selector1/1
  [CMBNE_SGNLS] -> Bus Selector8/1, Bus Selector6/1
  Bus Selector6/1 -> EPC_PV/1
  [CMBNE_SGNLS] -> Bus Selector7/1
  Bus Selector7/1 -> EPC_BESS/1
  Bus Selector8/1 -> Scope/1  "<Iabc>"
  Bus Selector8/4 -> Scope/4  "<Vabc_line>"
  Bus Selector8/2 -> Scope/2  "<Vabc_line>"
  Bus Selector8/3 -> Scope/3  "<Iabc>"
  Bus Selector9/1 -> SUBSTATION/1
  [CMBNE_SGNLS] -> Bus Selector9/1

== system BANSHEE/SC_ctrl/TestSeq ==
  TestData : Inport
  Bus Selector : BusSelector  OutputSignals=TestSeq.TimeStamp,TestSeq.fault_location_1,TestSeq.fault_location_2,TestSeq.fault_location_3,TestSeq.fault_location_4,TestSeq.fault_location_5,TestSeq.Cut_Grid_Power,TestSeq.Irradiance,TestSeq.motor_1,TestSeq.motor_2,TestSeq.Test3
  Display : Display
  Scope : Scope  NumInputPorts=10
  wires:
  TestData/1 -> Bus Selector/1
  Bus Selector/1 -> Display/1  "<TimeStamp>"
  Bus Selector/6 -> Scope/5  "<fault_location_5>"
  Bus Selector/5 -> Scope/4  "<fault_location_4>"
  Bus Selector/10 -> Scope/9  "<motor_2>"
  Bus Selector/2 -> Scope/1  "<fault_location_1>"
  Bus Selector/3 -> Scope/2  "<fault_location_2>"
  Bus Selector/8 -> Scope/7  "<Irradiance>"
  Bus Selector/9 -> Scope/8  "<motor_1>"
  Bus Selector/4 -> Scope/3  "<fault_location_3>"
  Bus Selector/7 -> Scope/6  "<Cut_Grid_Power>"
  Bus Selector/11 -> Scope/10  "<Test3>"

== system BANSHEE/SC_ctrl/Woodward ==
  16Din/16Dout GR3 : Subsystem
  Bus Creator2 : BusCreator  Inputs=1
  IOctrl : Outport
  wires:
  16Din/16Dout GR3/1(Dout) -> Bus Creator2/1  "16 DOUT GR3"
  Bus Creator2/1 -> IOctrl/1  "IO ctrl"

== system BANSHEE/SM_UtilityService/Banshee_HWCtrl_IOs ==
  note: When the system uses the simulated
      | Secondary Controller the digital I/O
      | should be disabled.
  note: Copyright (c) 2016 Massachusetts Institute of Technology
      | Permission is hereby granted, free of charge, to any person obtaining a copy of this software and associated documentation files (the "Software"), to deal
      | in the Software without restriction, including without limitation the rights to use, copy, modify, merge, publish, distribute, sublicense, and/or sell copies of the
      | Software, and to permit persons to whom the Software is furnished to do so, subject to the following conditions:
      |
      | THE SOFTWARE IS PROVIDED "AS IS", WITHOUT WARRANTY OF ANY KIND, EXPRESS OR IMPLIED, INCLUDING BUT NOT LIMITED TO THE
      | WARRANTIES OF MERCHANTABILITY, FITNESS FOR A PARTICULAR PURPOSE AND NONINFRINGEMENT. IN NO EVENT SHALL THE AUTHORS
      | OR COPYRIGHT HOLDERS BE LIABLE FOR ANY CLAIM, DAMAGES OR OTHER LIABILITY, WHETHER IN AN ACTION OF CONTRACT, TORT OR
      | OTHERWISE, ARISING FROM, OUT OF OR IN CONNECTION WITH THE SOFTWARE OR THE USE OR OTHER DEALINGS IN THE SOFTWARE
  note: USE NEW  BITSTREAM
      | To use old bitstream, change Digital Output Channel from 13 to 9 inside
      | "SEL751_01_DigitalAnalog_IO_OpBlocks" block
  ScaledSignals : Inport
  CMBNE_SGNLS : Inport  Port=2
  DTT_like_Signal : Inport  Port=3
  Bus Creator : BusCreator  Inputs=4
  Bus Creator1 : BusCreator  Inputs=5
  Bus Creator2 : BusCreator  Inputs=5
  Bus Creator3 : BusCreator  Inputs=4
  Bus Selector1 : BusSelector  OutputSignals=MCB_CB_Status
  Bus Selector2 : BusSelector  OutputSignals=scaled_gcb_voltage,scaled_gcb_current,scaled_mcb_voltage,scaled_mcb_current,scaled_speed
  Bus Selector3 : BusSelector  OutputSignals=NGCHP_ScaledSignals,Diesel_ScaledSignals,SEL751_ScaledSignals
  Bus Selector4 : BusSelector  OutputSignals=scaled_gcb_voltage,scaled_gcb_current,scaled_mcb_voltage,scaled_mcb_current,scaled_speed
  Bus Selector5 : BusSelector  OutputSignals=MCB_CB_Status
  Demux1 : Demux  Outputs=16
  GR1 B AIN (CH00-15) : Subsystem
  Memory1 : Memory
  OP5142EX1 Ctrl : rtio_opalrt_op5142ex1/OpCtrl OP5142EX1  CtrlName='OP5142EX1 Ctrl'  boardid=1  BitstreamFilename=OP5142_1-EX-0000-2_3_5_87-16AI_48AO_32DIO_16DO_16selDO_CD-FF-01.bin  numconfig=-1  mode=Slave  externalClock=off  decimRtsi=0  calibIO=off  SampleTime=0  loadinport=-1
  OpCtrl : rtio_opalrt_common/OpCtrl  CtrlName='OpCtrl'  boardid=0  BitstreamFilename=VC707_2-EX-0001-2_3_2_20-48AIO16DIO16DIOSel-02-01.bin  numconfig=-1  mode=Master  externalClock=off  decimRtsi=0  calibIO=off  SampleTime=0  loadinport=-1  BoardType=VC707  SecondaryPresent=off  sync_type=Audio
  SEL-2440 FAST-LOAD-SHEDDING AND CB STATUS : Subsystem
  SEL751_DigitalAnalog_IO_OpBlocks : Subsystem
  Woodward Inputs : Subsystem
  Woodward Outputs - Diesel - Gen2 : Subsystem
  Woodward Outputs - NGCHP - Gen1 : Subsystem
  WoodwardBias : Outport
  wires:
  Bus Creator/1 -> [WoodwardBias]
  Memory1/1 -> WoodwardBias/1
  Bus Selector1/1 -> Woodward Outputs - NGCHP - Gen1/1(Gen1 MCB Status)  "<MCB_CB_Status>"
  [NGCHP_ScaledSignals] -> Bus Selector1/1
  [WoodwardBias] -> Woodward Outputs - NGCHP - Gen1/2(WoodwardBias)
  Woodward Outputs - NGCHP - Gen1/5(Gen1 MCB) -> Bus Creator2/5  "MCB_Ctrl"
  Woodward Outputs - Diesel - Gen2/1(Digital Inputs) -> Bus Creator1/1  "DIN"
  Woodward Outputs - NGCHP - Gen1/4(Gen1 GCB) -> Bus Creator2/4  "GCB_Crtl"
  Woodward Outputs - NGCHP - Gen1/3(Gen1 Fuel Enable) -> Bus Creator2/3  "FuelEnable"
  Woodward Outputs - NGCHP - Gen1/2(Gen1 Gov and AVR) -> Bus Creator2/2  "Gov_and_AVR"
  Woodward Outputs - NGCHP - Gen1/1(Digital Inputs) -> Bus Creator2/1  "DIN"
  Bus Creator2/1 -> Bus Creator3/1  "NGCHP_Gen1"
  Bus Creator3/1 -> Memory1/1
  Bus Creator1/1 -> Bus Creator3/2  "Diesel_Gen2"
  Woodward Outputs - Diesel - Gen2/5(Gen2 MCB) -> Bus Creator1/5  "MCB_Ctrl"
  Woodward Outputs - Diesel - Gen2/4(Gen2 GCB) -> Bus Creator1/4  "GCB_Crtl"
  Woodward Outputs - Diesel - Gen2/3(Gen2 Fuel Enable) -> Bus Creator1/3  "FuelEnable"
  Woodward Outputs - Diesel - Gen2/2(Gen2 Gov and AVR) -> Bus Creator1/2  "Gov_and_AVR"
  [Diesel_ScaledSignals] -> Bus Selector5/1
  [WoodwardBias] -> Woodward Outputs - Diesel - Gen2/2(WoodwardBias)
  Bus Selector5/1 -> Woodward Outputs - Diesel - Gen2/1(Gen2 MCB Status)  "<MCB_CB_Status>"
  Demux1/4 -> Bus Creator/4  "gen2_AVR_bias"
  Demux1/3 -> Bus Creator/3  "gen2_GOV_bias"
  Demux1/2 -> Bus Creator/2  "gen1_AVR_bias"
  Demux1/1 -> Bus Creator/1  "gen1_GOV_bias"
  GR1 B AIN (CH00-15)/1(Out1) -> Demux1/1
  Bus Selector4/5 -> Woodward Inputs/10(MPU2_speed)  "<scaled_speed>"
  Bus Selector4/4 -> Woodward Inputs/9(Mains2_Current)  "<scaled_mcb_current>"
  Bus Selector4/3 -> Woodward Inputs/8(Mains2_Voltage)  "<scaled_mcb_voltage>"
  Bus Selector4/2 -> Woodward Inputs/7(Generator2_Current)  "<scaled_gcb_current>"
  Bus Selector4/1 -> Woodward Inputs/6(Generator2_Voltage)  "<scaled_gcb_voltage>"
  [Diesel_ScaledSignals] -> Bus Selector4/1
  Bus Selector2/1 -> Woodward Inputs/1(Generator1_Voltage)  "<scaled_gcb_voltage>"
  Bus Selector2/2 -> Woodward Inputs/2(Generator1_Current)  "<scaled_gcb_current>"
  Bus Selector2/3 -> Woodward Inputs/3(Mains1_Voltage)  "<scaled_mcb_voltage>"
  Bus Selector2/4 -> Woodward Inputs/4(Mains1_Current)  "<scaled_mcb_current>"
  Bus Selector2/5 -> Woodward Inputs/5(MPU1_speed)  "<scaled_speed>"
  [NGCHP_ScaledSignals] -> Bus Selector2/1
  Bus Selector3/2 -> [Diesel_ScaledSignals]  "<Diesel_ScaledSignals>"
  Bus Selector3/1 -> [NGCHP_ScaledSignals]  "<NGCHP_ScaledSignals>"
  ScaledSignals/1 -> Bus Selector3/1
  SEL751_DigitalAnalog_IO_OpBlocks/1(SEL751-01_LogicTrip) -> Bus Creator3/3  "SEL751_LogicTrip"
  Bus Selector3/3 -> [SEL751_ScaledSignals]  "<SEL751_ScaledSignals>"
  [SEL751_ScaledSignals] -> SEL751_DigitalAnalog_IO_OpBlocks/1(SEL751-01_ScaledSignals)
  CMBNE_SGNLS/1 -> SEL-2440 FAST-LOAD-SHEDDING AND CB STATUS/1(CMBNE_SGNLS)
  SEL-2440 FAST-LOAD-SHEDDING AND CB STATUS/1(SEL2440_FLS) -> Bus Creator3/4  "SEL2440_FLS"
  DTT_like_Signal/1 -> SEL751_DigitalAnalog_IO_OpBlocks/2(DTT_like_Signal)

== system BANSHEE/SM_UtilityService/Number of seconds of recording ==
  Compare To Constant1 : simulink/Logic and Bit Operations/Compare To Constant  relop=>=  const=time_s  OutDataTypeStr=boolean
  Increment : Subsystem
  Integrator : Integrator  ExternalReset=rising
  Memory : Memory
  Slope : Constant
  file suffix : Outport
  wires:
  Increment/1(Out1) -> file suffix/1
  Memory/1 -> Integrator/2
  Compare To Constant1/1 -> Increment/Trigger, Memory/1  "limit reached"
  Integrator/1 -> Compare To Constant1/1
  Slope/1 -> Integrator/1

== system BANSHEE/SM_UtilityService/TestSequenceCommands ==
  note: Copyright (c) 2016 Massachusetts Institute of Technology
      | Permission is hereby granted, free of charge, to any person obtaining a copy of this software and associated documentation files (the "Software"), to deal
      | in the Software without restriction, including without limitation the rights to use, copy, modify, merge, publish, distribute, sublicense, and/or sell copies of the
      | Software, and to permit persons to whom the Software is furnished to do so, subject to the following conditions:
      |
      | THE SOFTWARE IS PROVIDED "AS IS", WITHOUT WARRANTY OF ANY KIND, EXPRESS OR IMPLIED, INCLUDING BUT NOT LIMITED TO THE
      | WARRANTIES OF MERCHANTABILITY, FITNESS FOR A PARTICULAR PURPOSE AND NONINFRINGEMENT. IN NO EVENT SHALL THE AUTHORS
      | OR COPYRIGHT HOLDERS BE LIABLE FOR ANY CLAIM, DAMAGES OR OTHER LIABILITY, WHETHER IN AN ACTION OF CONTRACT, TORT OR
      | OTHERWISE, ARISING FROM, OUT OF OR IN CONNECTION WITH THE SOFTWARE OR THE USE OR OTHER DEALINGS IN THE SOFTWARE
  Add : Sum
  Bus Creator : BusCreator  Inputs=11
  Demux : Demux  Outputs=12
  Gain : Gain  Gain=2^16
  Modbus device : rtio_generic_modbus/Modbus device  conf_name=TestSequenceCmd_cfg.opal  conf_name_mask=TestSequenceCmd_cfg.xls  sample_time=Ts
  TestSeqData : Outport
  wires:
  Demux/12 -> Bus Creator/11  "Test3"
  Demux/3 -> Bus Creator/2  "fault_location_1"
  Demux/4 -> Bus Creator/3  "fault_location_2"
  Demux/5 -> Bus Creator/4  "fault_location_3"
  Demux/6 -> Bus Creator/5  "fault_location_4"
  Demux/7 -> Bus Creator/6  "fault_location_5"
  Demux/8 -> Bus Creator/7  "Cut_Grid_Power"
  Demux/9 -> Bus Creator/8  "Irradiance"
  Demux/10 -> Bus Creator/9  "motor_1"
  Add/1 -> Bus Creator/1  "TimeStamp"
  Demux/1 -> Add/1
  Demux/2 -> Gain/1
  Gain/1 -> Add/2
  Modbus device/1 -> Demux/1
  Demux/11 -> Bus Creator/10  "motor_2"
  Bus Creator/1 -> TestSeqData/1

== system BANSHEE/SM_UtilityService/Trigg_machine ==
  Write : Inport
  Odd : Inport  Port=2
  Even : Inport  Port=3
  Bitwise Operator : simulink/Logic and Bit Operations/Bitwise Operator  logicop=AND  UseBitMask=off  NumInputPorts=2  BitMask=bin2dec('11011001')  BitMaskRealWorld=Stored Integer
  Bitwise Operator1 : simulink/Logic and Bit Operations/Bitwise Operator  logicop=AND  UseBitMask=off  NumInputPorts=2  BitMask=bin2dec('11011001')  BitMaskRealWorld=Stored Integer
  Data Type Conversion : DataTypeConversion
  Data Type Conversion1 : DataTypeConversion
  Double2uint8 : DataTypeConversion
  Trig_odd : Outport
  Trig_even : Outport  Port=2
  wires:
  Bitwise Operator/1 -> Data Type Conversion/1
  Bitwise Operator1/1 -> Data Type Conversion1/1
  Even/1 -> Bitwise Operator1/2
  Data Type Conversion/1 -> Trig_odd/1
  Data Type Conversion1/1 -> Trig_even/1
  Odd/1 -> Bitwise Operator/1
  Write/1 -> Double2uint8/1
  Double2uint8/1 -> Bitwise Operator/2, Bitwise Operator1/1

== system BANSHEE/SM_UtilityService/isOddOrEven ==
  note: Effectuer la différence entre le nombre en entrée,
      | et sa moitié arrondie multipliée par 2.
  note: Si cette différence est égale à 0, c'est que le
      | nombre en entrée est pair, sinon c'est qu'il est impair.
  Index : Inport
  Compare To Zero : simulink/Logic and Bit Operations/Compare To Zero  relop=~=  OutDataTypeStr=boolean  ZeroCross=off
  Compare To Zero1 : simulink/Logic and Bit Operations/Compare To Zero  relop===  OutDataTypeStr=boolean  ZeroCross=off
  Constant3 : Constant  Value=2
  Divide : Product  Inputs=*/  OutDataTypeStr=double
  Produit : Product  Inputs=**  OutDataTypeStr=double
  Rounding Function : Rounding
  Sum : Sum  Inputs=|+-
  isOdd : Outport
  isEven : Outport  Port=2
  wires:
  Constant3/1 -> Divide/2, Produit/2
  Divide/1 -> Rounding Function/1
  Index/1 -> Divide/1, Sum/1
  Rounding Function/1 -> Produit/1
  Produit/1 -> Sum/2
  Sum/1 -> Compare To Zero/1, Compare To Zero1/1
  Compare To Zero/1 -> isOdd/1
  Compare To Zero1/1 -> isEven/1
